simulink model "MPC_MD_gaslift"  (R2023a)
settings: Solver=ode15s  StartTime=0.0  StopTime=par.simulation_time  FixedStep=par.sample_time  RelTol=1e-3
values from neighbouring files (symbols this model uses):
  A = blkdiag(plant_discrete.A, plant_output_disturbance.A)    [main_MPC_MD_gaslift.m]
  Bu = [plant_discrete.B; 0 0]    [main_MPC_MD_gaslift.m]
  Cm = [plant_discrete.C, plant_output_disturbance.C]    [main_MPC_MD_gaslift.m]
  par = function_parameters_MPC_MD_gaslift    [main_MPC_MD_gaslift.m]
  u0 = [operating_report.Inputs(1).u; par.pres]    [main_MPC_MD_gaslift.m]
  x0 = [operating_report.States(1).x; operating_report.States(2).x]    [main_MPC_MD_gaslift.m]
  y0 = operating_report.Outputs.y    [main_MPC_MD_gaslift.m]
undefined symbols (not defined in the file or in its folder): L, M
libraries: mpclib x1
settings Model: Creator=aslik  LastModifiedBy=aslik
settings DataIOCC: ExternalInput=getinputstruct(op_trim1)  InitialState=getstatestruct(op_trim1)  ReturnWorkspaceOutputs=off  DatasetSignalFormat=timetable

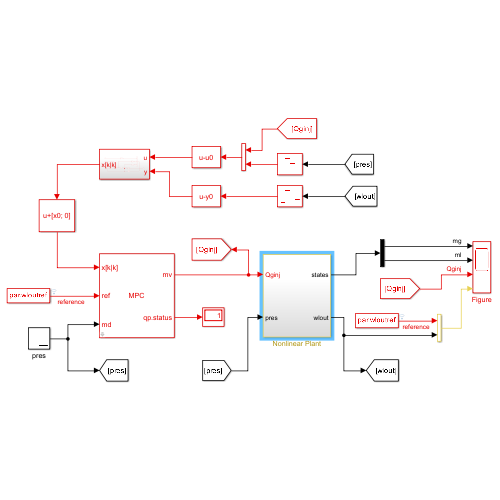
[thumbnail: Simulink's stored preview of the top-level diagram]
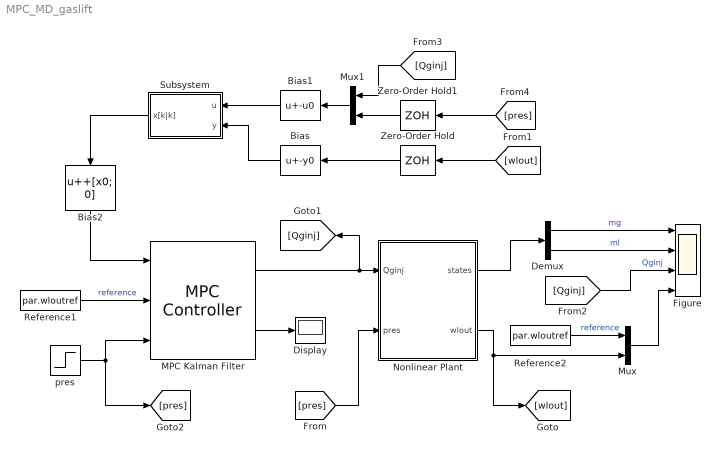
== system MPC_MD_gaslift ==
  Bias : Bias  Bias=-y0  SaturateOnIntegerOverflow=off
  Bias1 : Bias  Bias=-u0  SaturateOnIntegerOverflow=off
  Bias2 : Bias  Bias=+[x0; 0]  SaturateOnIntegerOverflow=off
  Demux : Demux  Outputs=2
  Display : Display
  Figure : Scope  NumInputPorts=4
  MPC Kalman Filter : mpclib/MPC Controller  mpcobj=mpcobj  x0=[]  is_multiple=0  enable_value=0  return_u0=off  updateMPCinCallerWorkspace=on  md_inport=on  mv_inport=off  uref_inport=off  return_cost=off  return_mvseq=off  return_qpstatus=on  return_xseq=off  return_state=off  return_ovseq=off  state_inport=on  umin_inport=off  umax_inport=off  ymin_inport=off  ymax_inport=off  cc_inport=off  ywt_inport=off  uwt_inport=off  duwt_inport=off  rhoeps_inport=off  pm_inport=off  MaximumP=10  HorizonChoice=FixedHorizon  n_ts=0.1  n_p=50  n_mv=1  n_md=1  n_ud=0  n_mo=1  n_uo=0  BlockDataType=double  SampleTimeInherited=off  switch_inport=off
  Mux : Mux  Inputs=2
  Mux1 : Mux  Inputs=2
  Nonlinear Plant : Subsystem
  Reference1 : Constant  Value=par.wloutref  SampleTime=0
  Reference2 : Constant  Value=par.wloutref  SampleTime=0
  Subsystem : Subsystem
  Zero-Order Hold : ZeroOrderHold  SampleTime=par.sample_time
  Zero-Order Hold1 : ZeroOrderHold  SampleTime=par.sample_time
  pres : Step  Time=20  Before=par.pres  After=par.pres_final  SampleTime=0
  wires:
  Demux/2 -> Figure/2  "ml"
  Demux/1 -> Figure/1  "mg"
  MPC Kalman Filter/1 -> Nonlinear Plant/1(Qginj), [Qginj]
  Nonlinear Plant/1(states) -> Demux/1
  Reference1/1 -> MPC Kalman Filter/2  "reference"
  MPC Kalman Filter/2 -> Display/1
  [Qginj] -> Figure/3  "Qginj"
  Bias2/1 -> MPC Kalman Filter/1
  pres/1 -> [pres], MPC Kalman Filter/3
  Mux/1 -> Figure/4
  Reference2/1 -> Mux/1  "reference"
  [wlout] -> Zero-Order Hold/1
  Zero-Order Hold/1 -> Bias/1
  Subsystem/1(x[k|k]) -> Bias2/1
  Bias1/1 -> Subsystem/1(u)
  [Qginj] -> Mux1/1
  Bias/1 -> Subsystem/2(y)
  Mux1/1 -> Bias1/1
  [pres] -> Zero-Order Hold1/1
  [pres] -> Nonlinear Plant/2(pres)
  Zero-Order Hold1/1 -> Mux1/2
  Nonlinear Plant/2(wlout) -> Mux/2, [wlout]

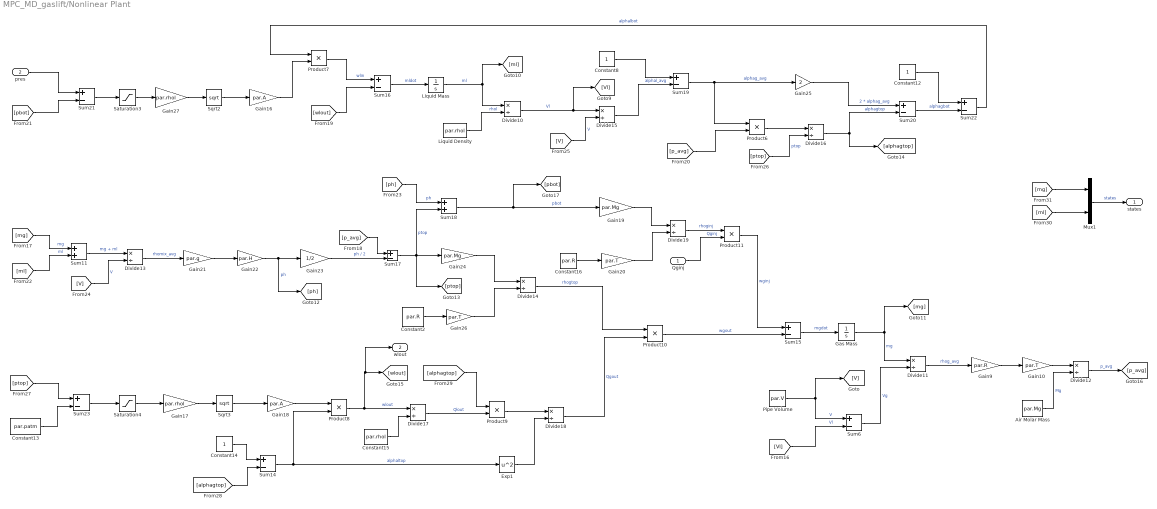
== system MPC_MD_gaslift/Nonlinear Plant ==
  Qginj : Inport
  pres : Inport  Port=2
  Air Molar Mass : Constant  Value=par.Mg  OutDataTypeStr=double
  Constant12 : Constant  OutDataTypeStr=double
  Constant13 : Constant  Value=par.patm  OutDataTypeStr=double
  Constant14 : Constant  OutDataTypeStr=double
  Constant15 : Constant  Value=par.rhol  OutDataTypeStr=double
  Constant16 : Constant  Value=par.R  OutDataTypeStr=double
  Constant2 : Constant  Value=par.R  OutDataTypeStr=double
  Constant8 : Constant  OutDataTypeStr=double
  Divide{10..19} (10 alike) : Product  Inputs=*/
  Exp1 : Math  Operator=square
  Gain10 : Gain  Gain=par.T
  Gain16 : Gain  Gain=par.A
  Gain17 : Gain  Gain=par.rhol
  Gain18 : Gain  Gain=par.A
  Gain19 : Gain  Gain=par.Mg
  Gain20 : Gain  Gain=par.T
  Gain21 : Gain  Gain=par.g
  Gain22 : Gain  Gain=par.H
  Gain23 : Gain  Gain=1/2
  Gain24 : Gain  Gain=par.Mg
  Gain25 : Gain  Gain=2
  Gain26 : Gain  Gain=par.T
  Gain27 : Gain  Gain=par.rhol
  Gain9 : Gain  Gain=par.R
  "Gas Mass " : Integrator  InitialCondition=x0(1)  LowerSaturationLimit=0  ContinuousStateAttributes='mg'
  Liquid Density : Constant  Value=par.rhol  OutDataTypeStr=double
  Liquid Mass : Integrator  InitialCondition=x0(2)  LowerSaturationLimit=0  ContinuousStateAttributes='ml'
  Mux1 : Mux  Inputs=2
  Pipe Volume : Constant  Value=par.V  OutDataTypeStr=double
  Product{6..11} (6 alike) : Product
  Saturation3 : Saturate  UpperLimit=inf  LowerLimit=0
  Saturation4 : Saturate  UpperLimit=inf  LowerLimit=0
  Sqrt2 : Sqrt
  Sqrt3 : Sqrt
  Sum11 : Sum
  Sum{6,14..17,19..23} (10 alike) : Sum  Inputs=+-
  Sum18 : Sum
  states : Outport
  wlout : Outport  Port=2
  wires:
  Sum11/1 -> Divide13/1  "mg + ml"
  Gain20/1 -> Divide19/2
  "Gas Mass "/1 -> [mg], Divide11/1  "mg"
  Product10/1 -> Sum15/2  "wgout"
  Product7/1 -> Sum16/1  "wlin"
  Gain18/1 -> Product8/1
  [wlout] -> Sum16/2
  [V] -> Divide13/2  "V"
  Product8/1 -> wlout/1, [wlout], Divide17/1  "wlout"
  Divide12/1 -> [p_avg]  "p_avg"
  Sum21/1 -> Saturation3/1
  Pipe Volume/1 -> [V], Sum6/1  "V"
  Gain10/1 -> Divide12/1
  [p_avg] -> Product6/2
  Sum14/1 -> Product8/2, Exp1/1  "alphaltop"
  Sum17/1 -> Gain24/1, Sum18/2, [ptop]  "ptop"
  Gain19/1 -> Divide19/1
  Divide10/1 -> Divide15/1, [Vl]  "Vl"
  Constant16/1 -> Gain20/1
  [ptop] -> Sum23/1
  Gain17/1 -> Sqrt3/1
  [V] -> Divide15/2  "V"
  Divide17/1 -> Product9/2  "Qlout"
  Sum16/1 -> Liquid Mass/1  "mldot"
  Sum22/1 -> Product7/1  "alphalbot"
  Sqrt2/1 -> Gain16/1
  [ml] -> Sum11/2  "ml"
  [alphagtop] -> Sum14/2
  [mg] -> Sum11/1  "mg"
  Constant13/1 -> Sum23/2
  Liquid Mass/1 -> [ml], Divide10/1  "ml"
  Sum6/1 -> Divide11/2  "Vg"
  Gain22/1 -> [ph], Gain23/1  "ph"
  Saturation4/1 -> Gain17/1
  Sum18/1 -> [pbot], Gain19/1  "pbot"
  Divide19/1 -> Product11/1  "rhoginj"
  Product9/1 -> Divide18/1
  Air Molar Mass/1 -> Divide12/2  "Mg"
  Sum20/1 -> Sum22/2  "alphagbot"
  [ptop] -> Divide16/2  "ptop"
  Gain21/1 -> Gain22/1
  Divide15/1 -> Sum19/2  "alphal_avg"
  Product11/1 -> Sum15/1  "wginj"
  Sum19/1 -> Product6/1, Gain25/1  "alphag_avg"
  Liquid Density/1 -> Divide10/2  "rhol"
  Sqrt3/1 -> Gain18/1
  Constant8/1 -> Sum19/1
  Constant2/1 -> Gain26/1
  [pbot] -> Sum21/2
  Divide16/1 -> [alphagtop], Sum20/2  "alphagtop"
  Gain25/1 -> Sum20/1  "2 * alphag_avg"
  Exp1/1 -> Divide18/2
  Gain26/1 -> Divide14/2
  Gain27/1 -> Sqrt2/1
  [ph] -> Sum18/1  "ph"
  Constant14/1 -> Sum14/1
  Divide13/1 -> Gain21/1  "rhomix_avg"
  Gain9/1 -> Gain10/1
  Gain16/1 -> Product7/2
  pres/1 -> Sum21/1
  Divide11/1 -> Gain9/1  "rhog_avg"
  Saturation3/1 -> Gain27/1
  Divide18/1 -> Product10/2  "Qgout"
  [p_avg] -> Sum17/1
  Gain24/1 -> Divide14/1
  Product6/1 -> Divide16/1
  Sum15/1 -> "Gas Mass "/1  "mgdot"
  Gain23/1 -> Sum17/2  "ph / 2"
  Qginj/1 -> Product11/2  "Qginj"
  Divide14/1 -> Product10/1  "rhogtop"
  Sum23/1 -> Saturation4/1
  Constant15/1 -> Divide17/2
  Constant12/1 -> Sum22/1
  [Vl] -> Sum6/2  "Vl"
  [alphagtop] -> Product9/1
  Mux1/1 -> states/1  "states"
  [mg] -> Mux1/1
  [ml] -> Mux1/2

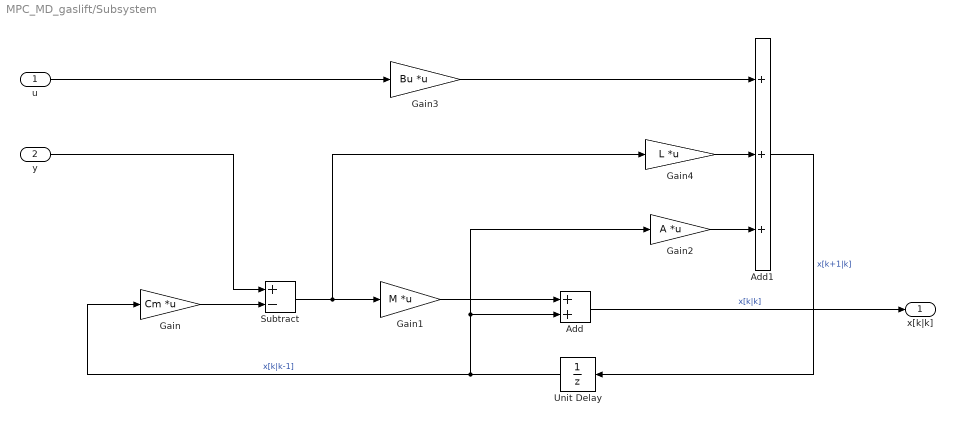
== system MPC_MD_gaslift/Subsystem ==
  u : Inport
  y : Inport  Port=2
  Add : Sum
  Add1 : Sum  Inputs=+++
  Gain : Gain  Gain=Cm  Multiplication=Matrix(K*u)
  Gain1 : Gain  Gain=M  Multiplication=Matrix(K*u)
  Gain2 : Gain  Gain=A  Multiplication=Matrix(K*u)
  Gain3 : Gain  Gain=Bu  Multiplication=Matrix(K*u)
  Gain4 : Gain  Gain=L  Multiplication=Matrix(K*u)
  Subtract : Sum  Inputs=+-
  Unit Delay : UnitDelay  InitialCondition=zeros(3,1)  SampleTime=par.sample_time  HasFrameUpgradeWarning=on
  x[k|k] : Outport  VectorParamsAs1DForOutWhenUnconnected=off
  wires:
  Unit Delay/1 -> Gain/1, Gain2/1, Add/2  "x[k|k-1]"
  Gain1/1 -> Add/1
  Add1/1 -> Unit Delay/1  "x[k+1|k]"
  Add/1 -> x[k|k]/1  "x[k|k]"
  Gain/1 -> Subtract/2
  Gain4/1 -> Add1/2
  Gain2/1 -> Add1/3
  Gain3/1 -> Add1/1
  u/1 -> Gain3/1
  y/1 -> Subtract/1
  Subtract/1 -> Gain4/1, Gain1/1
